simulink model "part1"  (R2024a)
settings: Solver=FixedStepAuto  StartTime=0.0  StopTime=2*10e4  FixedStep=0.001  RelTol=1e-3
PreLoadFcn:
  | k0 = 0.25;
  | k1 = 1;
  | a0 = 2;
  | a1 = 4;
  | b0 = 3;
  | b1 = 2;
  | theta = [k0 - a0; k1 - a1; b0; b1];
  | A0 = [-k1 1; -k0 0];
  | A = [-a1 1; -a1 0];
  | b = [b1; b0];
settings Model: Creator=ventus  LastModifiedBy=ventus

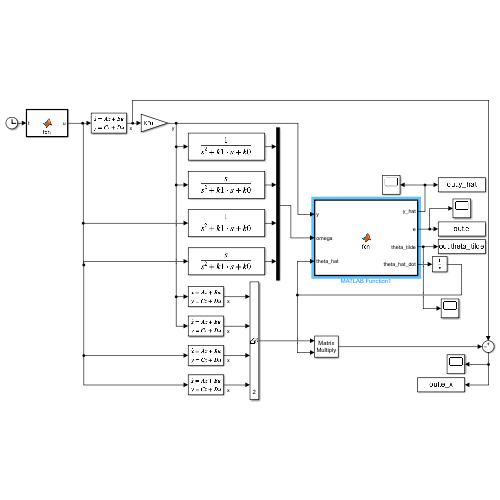
[thumbnail: Simulink's stored preview of the top-level diagram]
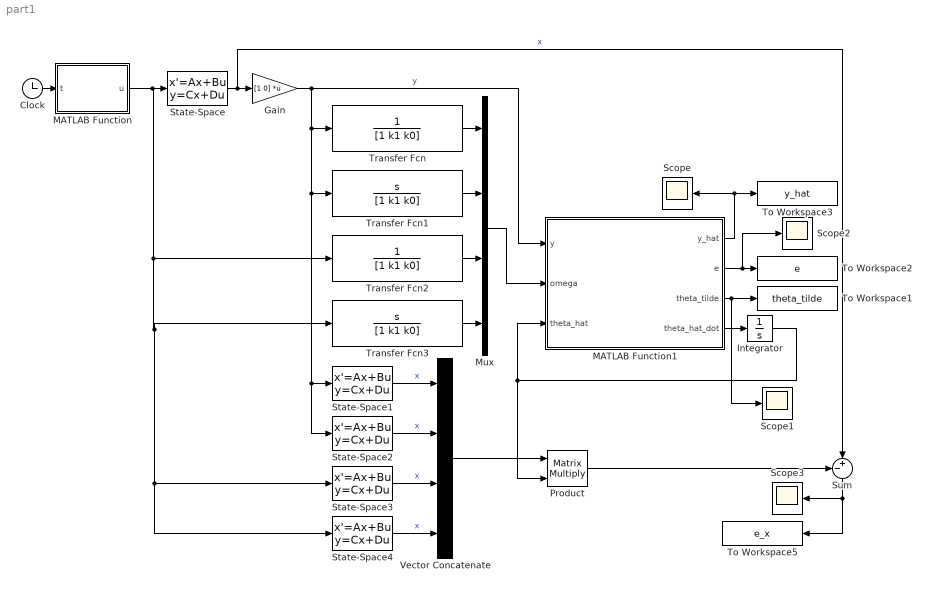
== system part1 ==
  Clock : Clock
  Gain : Gain  Gain=[1 0]  Multiplication=Matrix(K*u)
  Integrator : Integrator  InitialCondition=[0; 0; 0; 0]
  MATLAB Function : MATLAB Function  TreatAsAtomicUnit=on
  MATLAB Function1 : MATLAB Function  TreatAsAtomicUnit=on
  Mux : Mux
  Product : Product  Multiplication=Matrix(*)
  Scope{,1..3} (4 alike) : Scope
  State-Space : StateSpace  A=A  B=b  C=eye(2)  D=[0; 0]  InitialCondition=[0; 0]
  State-Space1 : StateSpace  A=A0  B=[0; 1]  C=eye(2)  D=[0; 0]  InitialCondition=[0; 0]
  State-Space2 : StateSpace  A=A0  B=[1; 0]  C=eye(2)  D=[0; 0]  InitialCondition=[0; 0]
  State-Space3 : StateSpace  A=A0  B=[0; 1]  C=eye(2)  D=[0; 0]  InitialCondition=[0; 0]
  State-Space4 : StateSpace  A=A0  B=[1; 0]  C=eye(2)  D=[0; 0]  InitialCondition=[0; 0]
  Sum : Sum  Inputs=-+|
  To Workspace1 : ToWorkspace  VariableName=theta_tilde  SaveFormat=Timeseries  SampleTime=-1
  To Workspace2 : ToWorkspace  VariableName=e  SaveFormat=Timeseries  SampleTime=-1
  To Workspace3 : ToWorkspace  VariableName=y_hat  SaveFormat=Timeseries  SampleTime=-1
  To Workspace5 : ToWorkspace  VariableName=e_x  SaveFormat=Timeseries  SampleTime=-1
  Transfer Fcn : TransferFcn  Denominator=[1 k1 k0]
  Transfer Fcn1 : TransferFcn  Numerator=[1 0]  Denominator=[1 k1 k0]
  Transfer Fcn2 : TransferFcn  Denominator=[1 k1 k0]
  Transfer Fcn3 : TransferFcn  Numerator=[1 0]  Denominator=[1 k1 k0]
  Vector Concatenate : Concatenate  NumInputs=4  Mode=Multidimensional array  ConcatenateDimension=2
  wires:
  State-Space/1 -> Sum/2, Gain/1  "x"
  Gain/1 -> Transfer Fcn/1, Transfer Fcn1/1, State-Space2/1, State-Space1/1, MATLAB Function1/1(y)  "y"
  MATLAB Function/1(u) -> State-Space3/1, State-Space4/1, Transfer Fcn3/1, Transfer Fcn2/1, State-Space/1
  Transfer Fcn3/1 -> Mux/4
  Transfer Fcn/1 -> Mux/1
  Transfer Fcn1/1 -> Mux/2
  Transfer Fcn2/1 -> Mux/3
  Mux/1 -> MATLAB Function1/2(omega)
  MATLAB Function1/4(theta_hat_dot) -> Integrator/1
  Integrator/1 -> Product/2, MATLAB Function1/3(theta_hat)
  State-Space1/1 -> Vector Concatenate/1  "x"
  State-Space4/1 -> Vector Concatenate/4  "x"
  State-Space3/1 -> Vector Concatenate/3  "x"
  State-Space2/1 -> Vector Concatenate/2  "x"
  Vector Concatenate/1 -> Product/1
  Product/1 -> Sum/1
  MATLAB Function1/3(theta_tilde) -> To Workspace1/1, Scope1/1
  MATLAB Function1/2(e) -> To Workspace2/1, Scope2/1
  MATLAB Function1/1(y_hat) -> To Workspace3/1, Scope/1
  Sum/1 -> To Workspace5/1, Scope3/1
  Clock/1 -> MATLAB Function/1(t)

== matlab function part1/MATLAB Function1 ==
  data: y input size=1; y_hat output size=1; omega input size=4; theta_hat input size=4; e output size=1; theta_tilde output size=4; theta_hat_dot output size=4
function [y_hat, e, theta_tilde, theta_hat_dot] = fcn(y, omega, theta_hat)    
    gamma = 3;

    a1 = 4;
    a0 = 2;
    
    b1 = 2;
    b0 = 3;

    k1 = 1;
    k0 = 0.25;

    theta = [k0 - a0; k1 - a1; b0; b1];

    y_hat = theta_hat' * omega;
    
    theta_tilde = theta - theta_hat;
    e = y - y_hat;
    theta_hat_dot = gamma * omega * e;

== matlab function part1/MATLAB Function ==
  data: t input; u output
function u = fcn(t)

u = 10*sin(t) + 5*cos(2*t) + 4*cos(4*t) + 3*cos(8*t);
%u = 10*sin(t);
